simulink model "Final_project"  (R2018a)
settings: Solver=FixedStepDiscrete  StartTime=0.0  StopTime=10.0  FixedStep=0.0005  RelTol=1e-3  EnableMultiTasking=on
InitFcn:
  | parameters
  | mbd_s32k14_consistency_checks(bdroot(gcs));
  | LinearVehicleGains
values from neighbouring files (symbols this model uses):
  Ak = 100    [parameters_template.m]
  b = 200    [parameters_template.m]
  base_ids = [10, 20, 30, 40, 50, 60]    [parameters_template.m]
  dT = 0.01    [parameters_template.m]
  H = 10    [ACCLogic_TestCase1.m]    (also in ACCLogic_TestCase2.m; parameters_template.m = 20)
  m = 2000    [parameters_template.m]
  n_desired = 0    [parameters_template.m]
  R = 1/5    (= 0.2)    [LinearVehicleGains.m]    (also in parameters_template.m)
  S_Kd1 = 0.0875    [parameters_template.m]
  S_Kd2 = 165    [parameters_template.m]
  S_Kp1 = 13.4    [parameters_template.m]
  S_Kp2 = 1473.5    [parameters_template.m]
  V_Ki = 50    [parameters_template.m]
  V_Kp = 5000    [parameters_template.m]
undefined symbols (not defined in the file or in its folder): DiscIntNeverNeededParam, LQFP
libraries: mbd_s32k14_ec_toolbox x54, simulink x21, xpcutilitieslib x15, Veh_Sim x9
(part 2 of 2)

== system Final_project/High Level Design/Outputs/write torque ==
  Reaction Torque : Inport  OutDataTypeStr=single
  Constant : Constant  Value=0  OutDataTypeStr=single
  Data Type Conversion : DataTypeConversion  OutDataTypeStr=single
  FTM_PWM_Config : mbd_s32k14_ec_toolbox/Motor Control Blocks/FTM Blocks/FTM_PWM_Config  Priority=1  ftmModule=0  ftmMode=Edge-Aligned PWM  ftmSourceClock=80 MHz  chan0En=on  chan0Type=Independent  chan2En=off  chan2Type=Independent  chan4En=off  chan4Type=Independent  chan6En=off  chan6Type=Independent  ftmPwmUnits=Hz  outFrequency=20000  ftmPeriod=4000  ftmPrescaler=Divide by 1  deadtimeUnits=Nanoseconds  deadtimeNs=0  deadtimeTicks=0  deadtimePrescaler=Divide by 1  dutyCycleCh0=0.25  dutyCycleCh1=0.25  dutyCycleCh2=0.25  dutyCycleCh3=0.25  dutyCycleCh4=0.25  dutyCycleCh5=0.25  dutyCycleCh6=0.25  dutyCycleCh7=0.25  dutyCycleSim=off  startAfterInit=on  showAdvOpt=on  pinFtmCh0=PTB12: [FTM0_CH0 | FTM Channel]  pinFtmCh1=None  pinPolCh0=Active High  pinPolCh1=Main duplicated  outputLevel0=High-true pulses  outputLevel1=High-true pulses  pinFtmCh2=PTB14: [FTM0_CH2 | FTM Channel]  pinFtmCh3=None  pinPolCh2=Active Low  pinPolCh3=Main duplicated  outputLevel2=High-true pulses  outputLevel3=High-true pulses  pinFtmCh4=PTB4: [FTM0_CH4 | FTM Channel]  pinFtmCh5=None  pinPolCh4=Active Low  pinPolCh5=Main duplicated  outputLevel4=Low-true pulses  outputLevel5=Low-true pulses  pinFtmCh6=PTA17: [FTM0_CH6 | FTM Channel]  pinFtmCh7=None  pinPolCh6=Active Low  pinPolCh7=Main duplicated  outputLevel6=High-true pulses  outputLevel7=High-true pulses  initTrigger=off  chTrigger0=off  chTrigger1=off  chTrigger2=off  chTrigger3=off  chTrigger4=off  chTrigger5=off  chTrigger6=off  chTrigger7=off  mcuTargetUpdate=on  pwmSyncTrg=Software trigger  pwmSyncHwRouting=TRGMUX_FTM7  pwmSyncTrg0=off  pwmSyncTrg1=off  pwmSyncTrg2=off  pwmSyncAutoClear=on  pwmSyncMinLoad=on  pwmSyncMaxLoad=on  pwmSyncInvert=System Clock  pwmSyncOutControl=System Clock  pwmSyncOutMask=System Clock  pwmSyncCounterInitial=System Clock  pwmSyncPoints=Update now  reloadEnable=off  reloadPriority=15  reloadHalfCycle=off  reloadHCR=0  reloadFrequency=0  chnMatch0=off  chnMatch1=off  chnMatch2=off  chnMatch3=off  chnMatch4=off  chnMatch5=off  chnMatch6=off  chnMatch7=off  pwmFaultProtection=off  pwmFaultInterrupt=off  pwmFaultClearing=Fault control disabled  pwmFaultPinState=Safe Value  pwmFaultFilterValue=0  pwmFaultPriority=15  fault_disen_0=off  fault_filter_0=off  fault_polarity_0=Active High  fault_disen_1=off  fault_filter_1=off  fault_polarity_1=Active high  fault_disen_2=off  fault_filter_2=off  fault_polarity_2=Active high  fault_disen_3=off  fault_filter_3=off  fault_polarity_3=Active high  fault_pin_0=None  fault_pin_1=None  fault_pin_2=None  fault_pin_3=None
  Subsystem2 : Subsystem
  wires:
  Subsystem2/1(Out1) -> FTM_PWM_Config/1
  Constant/1 -> FTM_PWM_Config/2
  Data Type Conversion/1 -> Subsystem2/1(In1)
  Reaction Torque/1 -> Data Type Conversion/1

== system Final_project/High Level Design/Subsystem/Inner Loop PD Control ==
  In1 : Inport
  Discrete Derivative : simulink/Discrete/Discrete Derivative  gainval=1.0  ICPrevScaledInput=0.0  OutMin=[]  OutMax=[]  OutDataType=fixdt(1, 16)  OutScaling=2^-10  DoSatur=off
  Gain6 : Gain  Gain=S_Kp2
  Gain7 : Gain  Gain=S_Kd2
  Sum5 : Sum  Inputs=|++
  "Auto-steer torque, Nmm" : Outport
  wires:
  Gain7/1 -> Discrete Derivative/1
  Sum5/1 -> "Auto-steer torque, Nmm"/1  "Auto-steer torque, Nmm"
  Gain6/1 -> Sum5/2
  In1/1 -> Gain6/1, Gain7/1
  Discrete Derivative/1 -> Sum5/1

== system Final_project/High Level Design/Subsystem/Outer loop PD Control ==
  In1 : Inport
  Discrete Derivative : simulink/Discrete/Discrete Derivative  gainval=1.0  ICPrevScaledInput=0.0  OutMin=[]  OutMax=[]  OutDataType=fixdt(1, 16)  OutScaling=2^-10  DoSatur=off
  Gain2 : Gain  Gain=S_Kd1
  Gain3 : Gain  Gain=S_Kp1
  Sum1 : Sum  Inputs=|++
  delta : Outport
  wires:
  Sum1/1 -> delta/1  "delta"
  Gain3/1 -> Sum1/2
  In1/1 -> Gain3/1, Gain2/1
  Gain2/1 -> Discrete Derivative/1
  Discrete Derivative/1 -> Sum1/1

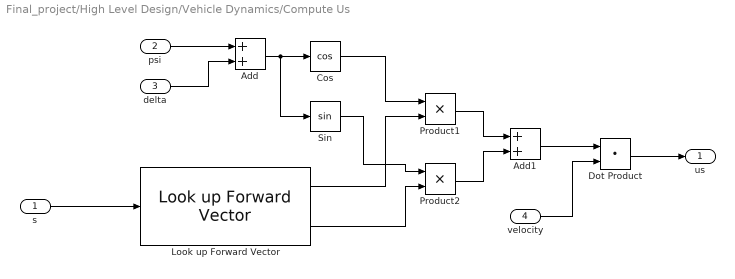
== system Final_project/High Level Design/Vehicle Dynamics/Compute Us ==
  s : Inport
  psi : Inport  Port=2
  delta : Inport  Port=3
  velocity : Inport  Port=4
  Add : Sum
  Add1 : Sum
  Cos : Trigonometry  Operator=cos
  Dot Product : DotProduct  InputSameDT=on  OutDataTypeStr=Inherit: Inherit via internal rule
  Look up Forward Vector : Veh_Sim/Look up Forward Vector  SystemSampleTime=-1
  Product1 : Product
  Product2 : Product
  Sin : Trigonometry
  us : Outport
  wires:
  Sin/1 -> Product2/1
  Add1/1 -> Dot Product/1
  Dot Product/1 -> us/1
  Cos/1 -> Product1/1
  delta/1 -> Add/2
  psi/1 -> Add/1
  Look up Forward Vector/1 -> Product1/2
  Look up Forward Vector/2 -> Product2/2
  Add/1 -> Sin/1, Cos/1
  Product1/1 -> Add1/1
  velocity/1 -> Dot Product/2
  Product2/1 -> Add1/2
  s/1 -> Look up Forward Vector/1

== system Final_project/High Level Design/Vehicle Dynamics/velocity calculation1 ==
  In1 : Inport
  Discrete-Time Integrator : DiscreteIntegrator  gainval=1  SampleTime=-1  ICPrevOutput=DiscIntNeverNeededParam  ICPrevScaledInput=DiscIntNeverNeededParam
  Gain : Gain  Gain=1/m
  Gain1 : Gain  Gain=b
  Subtract : Sum  Inputs=+-
  velocity : Outport
  wires:
  Subtract/1 -> Gain/1
  Discrete-Time Integrator/1 -> velocity/1, Gain1/1  "velocity"
  Gain1/1 -> Subtract/2
  Gain/1 -> Discrete-Time Integrator/1  "acceleration"
  In1/1 -> Subtract/1

== system Final_project/Serial Sim Out to Virtual Sim/UART Iteration/Resettable Subsystem ==
  Reset : ResetPort  DisableCoverage=on  ResetTriggerType=either
  Constant : Constant
  Delay : Delay  DelayLength=1
  Sum : Sum  Inputs=|++
  Out1 : Outport
  wires:
  Delay/1 -> Sum/1
  Constant/1 -> Sum/2
  Sum/1 -> Out1/1, Delay/1

== system Final_project/Can Network Inputs/Extract CAN data1/Data to s,n,psi,us /Switch Case Action Subsystem2 ==
  s,n : Inport
  Action Port : ActionPort  ActionType=then
  "Byte Unpacking " : xpcutilitieslib/Byte Unpacking   MaskUnpackedDataTypes={'single', 'single'}  MaskUnpackedDataSizes={[1], [1]}  MaskAlignment=1
      settings: SourceProductName=Simulink Real-Time  SourceProductBaseCode=XP
  s : Outport
  n : Outport  Port=2
  wires:
  s,n/1 -> "Byte Unpacking "/1
  "Byte Unpacking "/1 -> s/1
  "Byte Unpacking "/2 -> n/1

== system Final_project/Can Network Inputs/Extract CAN data1/Data to s,n,psi,us /Switch Case Action Subsystem3 ==
  psi,us : Inport
  Action Port : ActionPort  ActionType=elseif
  "Byte Unpacking " : xpcutilitieslib/Byte Unpacking   MaskUnpackedDataTypes={'single', 'single'}  MaskUnpackedDataSizes={[1], [1]}  MaskAlignment=1
      settings: SourceProductName=Simulink Real-Time  SourceProductBaseCode=XP
  psi : Outport
  us : Outport  Port=2
  wires:
  psi,us/1 -> "Byte Unpacking "/1
  "Byte Unpacking "/1 -> psi/1
  "Byte Unpacking "/2 -> us/1

== system Final_project/Can Network Inputs/Extract CAN data1/Data to s,n,psi,us 1/Switch Case Action Subsystem2 ==
  s,n : Inport
  Action Port : ActionPort  ActionType=then
  "Byte Unpacking " : xpcutilitieslib/Byte Unpacking   MaskUnpackedDataTypes={'single', 'single'}  MaskUnpackedDataSizes={[1], [1]}  MaskAlignment=1
      settings: SourceProductName=Simulink Real-Time  SourceProductBaseCode=XP
  s : Outport
  n : Outport  Port=2
  wires:
  s,n/1 -> "Byte Unpacking "/1
  "Byte Unpacking "/1 -> s/1
  "Byte Unpacking "/2 -> n/1

== system Final_project/Can Network Inputs/Extract CAN data1/Data to s,n,psi,us 1/Switch Case Action Subsystem3 ==
  psi,us : Inport
  Action Port : ActionPort  ActionType=elseif
  "Byte Unpacking " : xpcutilitieslib/Byte Unpacking   MaskUnpackedDataTypes={'single', 'single'}  MaskUnpackedDataSizes={[1], [1]}  MaskAlignment=1
      settings: SourceProductName=Simulink Real-Time  SourceProductBaseCode=XP
  psi : Outport
  us : Outport  Port=2
  wires:
  psi,us/1 -> "Byte Unpacking "/1
  "Byte Unpacking "/1 -> psi/1
  "Byte Unpacking "/2 -> us/1

== system Final_project/Can Network Inputs/Extract CAN data1/Data to s,n,psi,us 2/Switch Case Action Subsystem2 ==
  s,n : Inport
  Action Port : ActionPort  ActionType=then
  "Byte Unpacking " : xpcutilitieslib/Byte Unpacking   MaskUnpackedDataTypes={'single', 'single'}  MaskUnpackedDataSizes={[1], [1]}  MaskAlignment=1
      settings: SourceProductName=Simulink Real-Time  SourceProductBaseCode=XP
  s : Outport
  n : Outport  Port=2
  wires:
  s,n/1 -> "Byte Unpacking "/1
  "Byte Unpacking "/1 -> s/1
  "Byte Unpacking "/2 -> n/1

== system Final_project/Can Network Inputs/Extract CAN data1/Data to s,n,psi,us 2/Switch Case Action Subsystem3 ==
  psi,us : Inport
  Action Port : ActionPort  ActionType=elseif
  "Byte Unpacking " : xpcutilitieslib/Byte Unpacking   MaskUnpackedDataTypes={'single', 'single'}  MaskUnpackedDataSizes={[1], [1]}  MaskAlignment=1
      settings: SourceProductName=Simulink Real-Time  SourceProductBaseCode=XP
  psi : Outport
  us : Outport  Port=2
  wires:
  psi,us/1 -> "Byte Unpacking "/1
  "Byte Unpacking "/1 -> psi/1
  "Byte Unpacking "/2 -> us/1

== system Final_project/Can Network Inputs/Extract CAN data1/Data to s,n,psi,us 3/Switch Case Action Subsystem2 ==
  s,n : Inport
  Action Port : ActionPort  ActionType=then
  "Byte Unpacking " : xpcutilitieslib/Byte Unpacking   MaskUnpackedDataTypes={'single', 'single'}  MaskUnpackedDataSizes={[1], [1]}  MaskAlignment=1
      settings: SourceProductName=Simulink Real-Time  SourceProductBaseCode=XP
  s : Outport
  n : Outport  Port=2
  wires:
  s,n/1 -> "Byte Unpacking "/1
  "Byte Unpacking "/1 -> s/1
  "Byte Unpacking "/2 -> n/1

== system Final_project/Can Network Inputs/Extract CAN data1/Data to s,n,psi,us 3/Switch Case Action Subsystem3 ==
  psi,us : Inport
  Action Port : ActionPort  ActionType=elseif
  "Byte Unpacking " : xpcutilitieslib/Byte Unpacking   MaskUnpackedDataTypes={'single', 'single'}  MaskUnpackedDataSizes={[1], [1]}  MaskAlignment=1
      settings: SourceProductName=Simulink Real-Time  SourceProductBaseCode=XP
  psi : Outport
  us : Outport  Port=2
  wires:
  psi,us/1 -> "Byte Unpacking "/1
  "Byte Unpacking "/1 -> psi/1
  "Byte Unpacking "/2 -> us/1

== system Final_project/Can Network Inputs/Extract CAN data1/Data to s,n,psi,us 4/Switch Case Action Subsystem2 ==
  s,n : Inport
  Action Port : ActionPort  ActionType=then
  "Byte Unpacking " : xpcutilitieslib/Byte Unpacking   MaskUnpackedDataTypes={'single', 'single'}  MaskUnpackedDataSizes={[1], [1]}  MaskAlignment=1
      settings: SourceProductName=Simulink Real-Time  SourceProductBaseCode=XP
  s : Outport
  n : Outport  Port=2
  wires:
  s,n/1 -> "Byte Unpacking "/1
  "Byte Unpacking "/1 -> s/1
  "Byte Unpacking "/2 -> n/1

== system Final_project/Can Network Inputs/Extract CAN data1/Data to s,n,psi,us 4/Switch Case Action Subsystem3 ==
  psi,us : Inport
  Action Port : ActionPort  ActionType=elseif
  "Byte Unpacking " : xpcutilitieslib/Byte Unpacking   MaskUnpackedDataTypes={'single', 'single'}  MaskUnpackedDataSizes={[1], [1]}  MaskAlignment=1
      settings: SourceProductName=Simulink Real-Time  SourceProductBaseCode=XP
  psi : Outport
  us : Outport  Port=2
  wires:
  psi,us/1 -> "Byte Unpacking "/1
  "Byte Unpacking "/1 -> psi/1
  "Byte Unpacking "/2 -> us/1

== system Final_project/Can Network Inputs/Extract CAN data1/Data to s,n,psi,us 5/Switch Case Action Subsystem2 ==
  s,n : Inport
  Action Port : ActionPort  ActionType=then
  "Byte Unpacking " : xpcutilitieslib/Byte Unpacking   MaskUnpackedDataTypes={'single', 'single'}  MaskUnpackedDataSizes={[1], [1]}  MaskAlignment=1
      settings: SourceProductName=Simulink Real-Time  SourceProductBaseCode=XP
  s : Outport
  n : Outport  Port=2
  wires:
  s,n/1 -> "Byte Unpacking "/1
  "Byte Unpacking "/1 -> s/1
  "Byte Unpacking "/2 -> n/1

== system Final_project/Can Network Inputs/Extract CAN data1/Data to s,n,psi,us 5/Switch Case Action Subsystem3 ==
  psi,us : Inport
  Action Port : ActionPort  ActionType=elseif
  "Byte Unpacking " : xpcutilitieslib/Byte Unpacking   MaskUnpackedDataTypes={'single', 'single'}  MaskUnpackedDataSizes={[1], [1]}  MaskAlignment=1
      settings: SourceProductName=Simulink Real-Time  SourceProductBaseCode=XP
  psi : Outport
  us : Outport  Port=2
  wires:
  psi,us/1 -> "Byte Unpacking "/1
  "Byte Unpacking "/1 -> psi/1
  "Byte Unpacking "/2 -> us/1

== system Final_project/High Level Design/ACC State Logic/Speed Ctrl/PI ==
  Error : Inport
  Gain : Gain  Gain=V_Ki  SaturateOnIntegerOverflow=on  OutDataTypeStr=Inherit: Same as input  ParamDataTypeStr=Inherit: Same as input
  Gain1 : Gain  Gain=V_Kp  SaturateOnIntegerOverflow=on  OutDataTypeStr=Inherit: Same as input  ParamDataTypeStr=Inherit: Same as input
  My Discrete Integrator : Subsystem
  Sum : Sum  Inputs=|++  SaturateOnIntegerOverflow=on
  U : Outport
  wires:
  Sum/1 -> U/1
  Error/1 -> Gain1/1, Gain/1
  Gain1/1 -> Sum/2
  My Discrete Integrator/1(X) -> Sum/1
  Gain/1 -> My Discrete Integrator/1(X_dot)

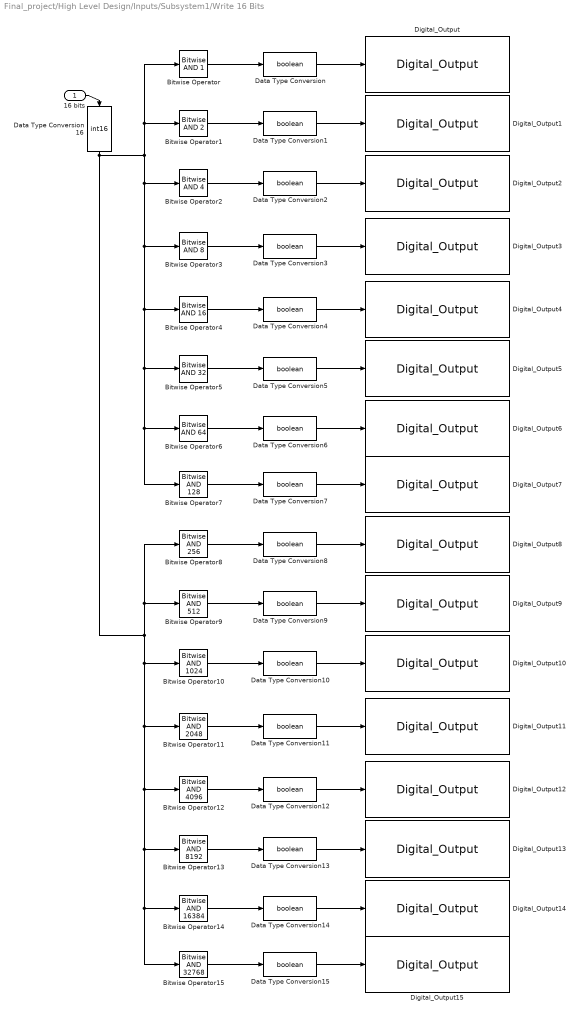
== system Final_project/High Level Design/Inputs/Subsystem1/Write 16 Bits ==
  16 bits : Inport
  Bitwise Operator : simulink/Logic and Bit Operations/Bitwise Operator  logicop=AND  UseBitMask=on  BitMask=1  BitMaskRealWorld=Stored Integer
  Bitwise Operator1 : simulink/Logic and Bit Operations/Bitwise Operator  logicop=AND  UseBitMask=on  BitMask=2  BitMaskRealWorld=Stored Integer
  Bitwise Operator10 : simulink/Logic and Bit Operations/Bitwise Operator  logicop=AND  UseBitMask=on  BitMask=1024  BitMaskRealWorld=Stored Integer
  Bitwise Operator11 : simulink/Logic and Bit Operations/Bitwise Operator  logicop=AND  UseBitMask=on  BitMask=2048  BitMaskRealWorld=Stored Integer
  Bitwise Operator12 : simulink/Logic and Bit Operations/Bitwise Operator  logicop=AND  UseBitMask=on  BitMask=4096  BitMaskRealWorld=Stored Integer
  Bitwise Operator13 : simulink/Logic and Bit Operations/Bitwise Operator  logicop=AND  UseBitMask=on  BitMask=8192  BitMaskRealWorld=Stored Integer
  Bitwise Operator14 : simulink/Logic and Bit Operations/Bitwise Operator  logicop=AND  UseBitMask=on  BitMask=16384  BitMaskRealWorld=Stored Integer
  Bitwise Operator15 : simulink/Logic and Bit Operations/Bitwise Operator  logicop=AND  UseBitMask=on  BitMask=32768  BitMaskRealWorld=Stored Integer
  Bitwise Operator2 : simulink/Logic and Bit Operations/Bitwise Operator  logicop=AND  UseBitMask=on  BitMask=4  BitMaskRealWorld=Stored Integer
  Bitwise Operator3 : simulink/Logic and Bit Operations/Bitwise Operator  logicop=AND  UseBitMask=on  BitMask=8  BitMaskRealWorld=Stored Integer
  Bitwise Operator4 : simulink/Logic and Bit Operations/Bitwise Operator  logicop=AND  UseBitMask=on  BitMask=16  BitMaskRealWorld=Stored Integer
  Bitwise Operator5 : simulink/Logic and Bit Operations/Bitwise Operator  logicop=AND  UseBitMask=on  BitMask=32  BitMaskRealWorld=Stored Integer
  Bitwise Operator6 : simulink/Logic and Bit Operations/Bitwise Operator  logicop=AND  UseBitMask=on  BitMask=64  BitMaskRealWorld=Stored Integer
  Bitwise Operator7 : simulink/Logic and Bit Operations/Bitwise Operator  logicop=AND  UseBitMask=on  BitMask=128  BitMaskRealWorld=Stored Integer
  Bitwise Operator8 : simulink/Logic and Bit Operations/Bitwise Operator  logicop=AND  UseBitMask=on  BitMask=256  BitMaskRealWorld=Stored Integer
  Bitwise Operator9 : simulink/Logic and Bit Operations/Bitwise Operator  logicop=AND  UseBitMask=on  BitMask=512  BitMaskRealWorld=Stored Integer
  Data Type Conversion{,1..15} (16 alike) : DataTypeConversion  OutDataTypeStr=boolean
  Data Type Conversion16 : DataTypeConversion  OutDataTypeStr=int16
  Digital_Output : mbd_s32k14_ec_toolbox/GPIO Blocks/Digital_Output  gpio_pin=PTD0: [PTD0 | Port D I/O]  drive_strength=Low
  Digital_Output1 : mbd_s32k14_ec_toolbox/GPIO Blocks/Digital_Output  gpio_pin=PTD1: [PTD1 | Port D I/O]  drive_strength=Low
  Digital_Output10 : mbd_s32k14_ec_toolbox/GPIO Blocks/Digital_Output  gpio_pin=PTD10: [PTD10 | Port D I/O]  drive_strength=Low
  Digital_Output11 : mbd_s32k14_ec_toolbox/GPIO Blocks/Digital_Output  gpio_pin=PTD11: [PTD11 | Port D I/O]  drive_strength=Low
  Digital_Output12 : mbd_s32k14_ec_toolbox/GPIO Blocks/Digital_Output  gpio_pin=PTD12: [PTD12 | Port D I/O]  drive_strength=Low
  Digital_Output13 : mbd_s32k14_ec_toolbox/GPIO Blocks/Digital_Output  gpio_pin=PTD13: [PTD13 | Port D I/O]  drive_strength=Low
  Digital_Output14 : mbd_s32k14_ec_toolbox/GPIO Blocks/Digital_Output  gpio_pin=PTD14: [PTD14 | Port D I/O]  drive_strength=Low
  Digital_Output15 : mbd_s32k14_ec_toolbox/GPIO Blocks/Digital_Output  gpio_pin=PTD15: [PTD15 | Port D I/O]  drive_strength=Low
  Digital_Output2 : mbd_s32k14_ec_toolbox/GPIO Blocks/Digital_Output  gpio_pin=PTD2: [PTD2 | Port D I/O]  drive_strength=Low
  Digital_Output3 : mbd_s32k14_ec_toolbox/GPIO Blocks/Digital_Output  gpio_pin=PTD3: [PTD3 | Port D I/O]  drive_strength=Low
  Digital_Output4 : mbd_s32k14_ec_toolbox/GPIO Blocks/Digital_Output  gpio_pin=PTD4: [PTD4 | Port D I/O]  drive_strength=Low
  Digital_Output5 : mbd_s32k14_ec_toolbox/GPIO Blocks/Digital_Output  gpio_pin=PTD5: [PTD5 | Port D I/O]  drive_strength=Low
  Digital_Output6 : mbd_s32k14_ec_toolbox/GPIO Blocks/Digital_Output  gpio_pin=PTD6: [PTD6 | Port D I/O]  drive_strength=Low
  Digital_Output7 : mbd_s32k14_ec_toolbox/GPIO Blocks/Digital_Output  gpio_pin=PTD7: [PTD7 | Port D I/O]  drive_strength=Low
  Digital_Output8 : mbd_s32k14_ec_toolbox/GPIO Blocks/Digital_Output  gpio_pin=PTD8: [PTD8 | Port D I/O]  drive_strength=Low
  Digital_Output9 : mbd_s32k14_ec_toolbox/GPIO Blocks/Digital_Output  gpio_pin=PTD9: [PTD9 | Port D I/O]  drive_strength=Low
  wires:
  Data Type Conversion4/1 -> Digital_Output4/1
  Data Type Conversion3/1 -> Digital_Output3/1
  Data Type Conversion2/1 -> Digital_Output2/1
  Data Type Conversion1/1 -> Digital_Output1/1
  Data Type Conversion/1 -> Digital_Output/1
  16 bits/1 -> Data Type Conversion16/1
  Bitwise Operator4/1 -> Data Type Conversion4/1
  Bitwise Operator3/1 -> Data Type Conversion3/1
  Bitwise Operator2/1 -> Data Type Conversion2/1
  Bitwise Operator1/1 -> Data Type Conversion1/1
  Bitwise Operator/1 -> Data Type Conversion/1
  Data Type Conversion5/1 -> Digital_Output5/1
  Bitwise Operator5/1 -> Data Type Conversion5/1
  Data Type Conversion6/1 -> Digital_Output6/1
  Bitwise Operator6/1 -> Data Type Conversion6/1
  Data Type Conversion7/1 -> Digital_Output7/1
  Bitwise Operator7/1 -> Data Type Conversion7/1
  Data Type Conversion12/1 -> Digital_Output12/1
  Data Type Conversion11/1 -> Digital_Output11/1
  Data Type Conversion10/1 -> Digital_Output10/1
  Data Type Conversion9/1 -> Digital_Output9/1
  Data Type Conversion8/1 -> Digital_Output8/1
  Bitwise Operator12/1 -> Data Type Conversion12/1
  Bitwise Operator11/1 -> Data Type Conversion11/1
  Bitwise Operator10/1 -> Data Type Conversion10/1
  Bitwise Operator9/1 -> Data Type Conversion9/1
  Bitwise Operator8/1 -> Data Type Conversion8/1
  Data Type Conversion13/1 -> Digital_Output13/1
  Bitwise Operator13/1 -> Data Type Conversion13/1
  Data Type Conversion14/1 -> Digital_Output14/1
  Bitwise Operator14/1 -> Data Type Conversion14/1
  Data Type Conversion15/1 -> Digital_Output15/1
  Bitwise Operator15/1 -> Data Type Conversion15/1
  Data Type Conversion16/1 -> Bitwise Operator2/1, Bitwise Operator3/1, Bitwise Operator4/1, Bitwise Operator5/1, Bitwise Operator6/1, Bitwise Operator7/1, Bitwise Operator1/1, Bitwise Operator/1, Bitwise Operator8/1, Bitwise Operator9/1, Bitwise Operator15/1, Bitwise Operator14/1, Bitwise Operator13/1, Bitwise Operator12/1, Bitwise Operator11/1, Bitwise Operator10/1

== system Final_project/High Level Design/Inputs/get wheel position/Subsystem ==
  In1 : Inport
  Data Type Conversion : DataTypeConversion  OutDataTypeStr=uint16
  Data Type Conversion1 : DataTypeConversion  OutDataTypeStr=int16
  Data Type Conversion2 : DataTypeConversion  OutDataTypeStr=single
  Gain : Gain  Gain=(3.14*2)/4000  ParamDataTypeStr=single
  Sum : Sum  Inputs=+-
  Sum1 : Sum  Inputs=|++  AccumDataTypeStr=single
  Unit Delay : UnitDelay  SampleTime=-1
  Unit Delay1 : UnitDelay  SampleTime=-1
  Out1 : Outport  OutDataTypeStr=single
  wires:
  Unit Delay/1 -> Sum/2
  Data Type Conversion/1 -> Sum/1, Unit Delay/1
  Sum1/1 -> Out1/1, Unit Delay1/1
  In1/1 -> Data Type Conversion/1
  Unit Delay1/1 -> Sum1/2
  Data Type Conversion1/1 -> Data Type Conversion2/1
  Sum/1 -> Data Type Conversion1/1
  Data Type Conversion2/1 -> Gain/1
  Gain/1 -> Sum1/1

== system Final_project/High Level Design/Outputs/Extract x,y,psi (Cars 1 - 6)/Extract x,y,psi ==
  s,n,psi,us : Inport
  Demux : Demux
  Mux : Mux  Inputs=3
  Terminator : Terminator
  s,n to x,y : Veh_Sim/s,n to x,y  SystemSampleTime=-1
  x,y,psi : Outport
  wires:
  Demux/1 -> s,n to x,y/1
  Demux/2 -> s,n to x,y/2
  s,n,psi,us/1 -> Demux/1
  s,n to x,y/1 -> Mux/1
  s,n to x,y/2 -> Mux/2
  Demux/3 -> Mux/3
  Mux/1 -> x,y,psi/1
  Demux/4 -> Terminator/1

== system Final_project/High Level Design/Outputs/Extract x,y,psi (Cars 1 - 6)/Extract x,y,psi1 ==
  s,n,psi,us : Inport
  Demux : Demux
  Mux : Mux  Inputs=3
  Terminator : Terminator
  s,n to x,y : Veh_Sim/s,n to x,y  SystemSampleTime=-1
  x,y,psi : Outport
  wires:
  Demux/1 -> s,n to x,y/1
  Demux/2 -> s,n to x,y/2
  s,n,psi,us/1 -> Demux/1
  s,n to x,y/1 -> Mux/1
  s,n to x,y/2 -> Mux/2
  Demux/3 -> Mux/3
  Mux/1 -> x,y,psi/1
  Demux/4 -> Terminator/1

== system Final_project/High Level Design/Outputs/Extract x,y,psi (Cars 1 - 6)/Extract x,y,psi2 ==
  s,n,psi,us : Inport
  Demux : Demux
  Mux : Mux  Inputs=3
  Terminator : Terminator
  s,n to x,y : Veh_Sim/s,n to x,y  SystemSampleTime=-1
  x,y,psi : Outport
  wires:
  Demux/1 -> s,n to x,y/1
  Demux/2 -> s,n to x,y/2
  s,n,psi,us/1 -> Demux/1
  s,n to x,y/1 -> Mux/1
  s,n to x,y/2 -> Mux/2
  Demux/3 -> Mux/3
  Mux/1 -> x,y,psi/1
  Demux/4 -> Terminator/1

== system Final_project/High Level Design/Outputs/Extract x,y,psi (Cars 1 - 6)/Extract x,y,psi3 ==
  s,n,psi,us : Inport
  Demux : Demux
  Mux : Mux  Inputs=3
  Terminator : Terminator
  s,n to x,y : Veh_Sim/s,n to x,y  SystemSampleTime=-1
  x,y,psi : Outport
  wires:
  Demux/1 -> s,n to x,y/1
  Demux/2 -> s,n to x,y/2
  s,n,psi,us/1 -> Demux/1
  s,n to x,y/1 -> Mux/1
  s,n to x,y/2 -> Mux/2
  Demux/3 -> Mux/3
  Mux/1 -> x,y,psi/1
  Demux/4 -> Terminator/1

== system Final_project/High Level Design/Outputs/Extract x,y,psi (Cars 1 - 6)/Extract x,y,psi4 ==
  s,n,psi,us : Inport
  Demux : Demux
  Mux : Mux  Inputs=3
  Terminator : Terminator
  s,n to x,y : Veh_Sim/s,n to x,y  SystemSampleTime=-1
  x,y,psi : Outport
  wires:
  Demux/1 -> s,n to x,y/1
  Demux/2 -> s,n to x,y/2
  s,n,psi,us/1 -> Demux/1
  s,n to x,y/1 -> Mux/1
  s,n to x,y/2 -> Mux/2
  Demux/3 -> Mux/3
  Mux/1 -> x,y,psi/1
  Demux/4 -> Terminator/1

== system Final_project/High Level Design/Outputs/Extract x,y,psi (Cars 1 - 6)/Extract x,y,psi5 ==
  s,n,psi,us : Inport
  Demux : Demux
  Mux : Mux  Inputs=3
  Terminator : Terminator
  s,n to x,y : Veh_Sim/s,n to x,y  SystemSampleTime=-1
  x,y,psi : Outport
  wires:
  Demux/1 -> s,n to x,y/1
  Demux/2 -> s,n to x,y/2
  s,n,psi,us/1 -> Demux/1
  s,n to x,y/1 -> Mux/1
  s,n to x,y/2 -> Mux/2
  Demux/3 -> Mux/3
  Mux/1 -> x,y,psi/1
  Demux/4 -> Terminator/1

== system Final_project/High Level Design/Outputs/write torque/Subsystem2 ==
  In1 : Inport
  Constant : Constant  Value=0.5  OutDataTypeStr=single
  Gain : Gain  Gain=3.162e-4
  Saturation : Saturate  UpperLimit=0.76  LowerLimit=0.24
  Sum : Sum  Inputs=|++
  Out1 : Outport
  wires:
  Constant/1 -> Sum/2
  Sum/1 -> Saturation/1
  In1/1 -> Gain/1
  Gain/1 -> Sum/1
  Saturation/1 -> Out1/1

== system Final_project/High Level Design/ACC State Logic/Speed Ctrl/PI/My Discrete Integrator ==
  X_dot : Inport
  Gain : Gain  Gain=dT  SaturateOnIntegerOverflow=on  OutDataTypeStr=Inherit: Same as input  ParamDataTypeStr=Inherit: Same as input
  Sum : Sum  Inputs=|++  SaturateOnIntegerOverflow=on  InputSameDT=on  OutDataTypeStr=Inherit: Same as first input
  Unit Delay : UnitDelay  SampleTime=-1
  X : Outport
  wires:
  Gain/1 -> Sum/1
  X_dot/1 -> Gain/1
  Sum/1 -> Unit Delay/1
  Unit Delay/1 -> Sum/2, X/1

== stateflow chart Final_project/High Level Design/ACC State Logic/Chart ==
  state MANUAL
    spd=false;
    pos=false;
    man=true;
  state POSITION
    spd=false;
    pos=true;
    man=false;
  state Speed
    spd=true;
    pos=false;
    man=false;
  (default) -> MANUAL : {spd =false;
      | pos=false;
      | man=true;}
  MANUAL -> Speed : [ACC_Enable==true]
  Speed -> POSITION [order 1] : [distance<=H&& distance~=0&&closest_car_spd<cruise_spd ]
  Speed -> MANUAL [order 2] : [ACC_Enable==false]
  POSITION -> Speed [order 1] : [closest_car_spd>cruise_spd+5||distance>H+5]
  POSITION -> MANUAL [order 2] : [ACC_Enable==0]
  data: man output boolean; ACC_Enable input boolean; distance input single; spd output boolean; pos output boolean; H parameter single; closest_car_spd input single; cruise_spd input single
